simulink library "inp"  (R2021b)
settings: Solver=VariableStepAuto  StartTime=0.0  StopTime=10.0  RelTol=1e-3
undefined symbols (not defined in the file): C_TASK_5MS_S, FALSE, KINP_AcoreReadyToSlp_flg_ovrdflg, KINP_AcoreReadyToSlp_flg_ovrdval, KINP_AllowMovThd_OTA_enum_ovrdflg, KINP_AllowMovThd_OTA_enum_ovrdval, KINP_APSAngleTarget_Deg_ovrdflg, KINP_APSAngleTarget_Deg_ovrdval, KINP_APSDecReq_mps2_ovrdflg, KINP_APSDecReq_mps2_ovrdval, KINP_APSDecReqA_flg_ovrdflg, KINP_APSDecReqA_flg_ovrdval, KINP_APSDFLL_cm_ovrdflg, KINP_APSDFLL_cm_ovrdval, KINP_APSDFLR_cm_ovrdflg, KINP_APSDFLR_cm_ovrdval, KINP_APSDRLL_cm_ovrdflg, KINP_APSDRLL_cm_ovrdval, KINP_APSDRLR_cm_ovrdflg, KINP_APSDRLR_cm_ovrdval, KINP_APSExitCondition_enum_ovrdflg, KINP_APSExitCondition_enum_ovrdval, KINP_APSHWVer_enum_ovrdflg, KINP_APSHWVer_enum_ovrdval, KINP_APSProgressPCT_pct_ovrdflg, KINP_APSProgressPCT_pct_ovrdval, KINP_APSReq_enum_ovrdflg, KINP_APSReq_enum_ovrdval, KINP_APSRQDisplay_enum_ovrdflg, KINP_APSRQDisplay_enum_ovrdval, KINP_APSRqEPASCtrl_flg_ovrdflg, KINP_APSRqEPASCtrl_flg_ovrdval, KINP_APSShiftPosnReq_enum_ovrdval, KINP_APSShiftPosnReq_enum_ovrflg, KINP_APSSpeedCMD_kph_ovrdval, KINP_APSSpeedCMD_kph_ovrflg, KINP_APSStaSystem_enum_ovrdflg, KINP_APSStaSystem_enum_ovrdval, KINP_APSSWVer_enum_ovrdflg, KINP_APSSWVer_enum_ovrdval, KINP_APSVMCReqA_flg_ovrdval, KINP_APSVMCReqA_flg_ovrflg, KINP_APSVRqEPASCtrl_flg_ovrdflg, KINP_APSVRqEPASCtrl_flg_ovrdval, KINP_AuxBattVolmV_mV_ovrdflg, KINP_AuxBattVolmV_mV_ovrdval, KINP_CAASSta_enum_ovrdflg, KINP_CAASSta_enum_ovrdval, KINP_CAASVMCReqA_flg_ovrdval, KINP_CAASVMCReqA_flg_ovrflg, KINP_Chime_enum_ovrdflg, KINP_Chime_enum_ovrdval, KINP_ClearDTCcmd_flg_ovrdflg, KINP_ClearDTCcmd_flg_ovrdval, KINP_EvccAplusPwrUpReq_flg_ovrdflg, KINP_EvccAplusPwrUpReq_flg_ovrdval, KINP_LFID_raw_ovrdval, KINP_LFID_raw_ovrflg, KINP_LRID_raw_ovrdval, KINP_MemOffsetAccX_raw16_ovrdflg ... (+118)
libraries: FVT_lib x942, hcu_lib x1
(part 21 of 31)

== system inp/INP/CAN3/SignalCheck/MCU_N_F1 ==
  BHAL_outputs : Inport
  inp_CanValid_bus : Inport  Port=2
  FrActvDmpDisabStaNidec : FVT_lib/inp/can_signal_template  SystemSampleTime=-1  VariantActivationTime=update diagram  Latency=0  AutoFrameSizeCalculation=off
      link override defval: Value=KINP_FrActvDmpDisabStaNidec_flg_defval
      link override ovrdflg: Value=KINP_FrActvDmpDisabStaNidec_flg_ovrdflg
      link override ovrdval: Value=KINP_FrActvDmpDisabStaNidec_flg_ovrdval
  FrEDUDrtStaNidec : FVT_lib/inp/can_signal_template  SystemSampleTime=-1  VariantActivationTime=update diagram  Latency=0  AutoFrameSizeCalculation=off
      link override defval: Value=KINP_FrEDUDrtStaNidec_flg_defval
      link override ovrdflg: Value=KINP_FrEDUDrtStaNidec_flg_ovrdflg
      link override ovrdval: Value=KINP_FrEDUDrtStaNidec_flg_ovrdval
  FrEDUOpratingStaNidec : FVT_lib/inp/can_signal_template  SystemSampleTime=-1  VariantActivationTime=update diagram  Latency=0  AutoFrameSizeCalculation=off
      link override defval: Value=KINP_FrEDUOpratingStaNidec_flg_defval
      link override ovrdflg: Value=KINP_FrEDUOpratingStaNidec_flg_ovrdflg
      link override ovrdval: Value=KINP_FrEDUOpratingStaNidec_flg_ovrdval
  FrEDURealTMTqNidec : FVT_lib/inp/can_signal_template  SystemSampleTime=-1  VariantActivationTime=update diagram  Latency=0  AutoFrameSizeCalculation=off
      link override defval: Value=KINP_FrEDURealTMTqNidec_Nm_defval
      link override ovrdflg: Value=KINP_FrEDURealTMTqNidec_Nm_ovrdflg
      link override ovrdval: Value=KINP_FrEDURealTMTqNidec_Nm_ovrdval
  FrEDURotateDirctionNidec : FVT_lib/inp/can_signal_template  SystemSampleTime=-1  VariantActivationTime=update diagram  Latency=0  AutoFrameSizeCalculation=off
      link override defval: Value=KINP_FrEDURotateDirctionNidec_enum_defval
      link override ovrdflg: Value=KINP_FrEDURotateDirctionNidec_enum_ovrdflg
      link override ovrdval: Value=KINP_FrEDURotateDirctionNidec_enum_ovrdval
  FrEDUTqReqFbkNidec : FVT_lib/inp/can_signal_template  SystemSampleTime=-1  VariantActivationTime=update diagram  Latency=0  AutoFrameSizeCalculation=off
      link override defval: Value=KINP_FrEDUTqReqFbkNidec_Nm_defval
      link override ovrdflg: Value=KINP_FrEDUTqReqFbkNidec_Nm_ovrdflg
      link override ovrdval: Value=KINP_FrEDUTqReqFbkNidec_Nm_ovrdval
  FrMCU1ChksumNidec : FVT_lib/inp/can_signal_template  SystemSampleTime=-1  VariantActivationTime=update diagram  Latency=0  AutoFrameSizeCalculation=off
      link override defval: Value=KINP_FrMCU1ChksumNidec_enum_defval
      link override ovrdflg: Value=KINP_FrMCU1ChksumNidec_enum_ovrdflg
      link override ovrdval: Value=KINP_FrMCU1ChksumNidec_enum_ovrdval
  FrMCU1RolCntNidec : FVT_lib/inp/can_signal_template  SystemSampleTime=-1  VariantActivationTime=update diagram  Latency=0  AutoFrameSizeCalculation=off
      link override defval: Value=KINP_FrMCU1RolCntNidec_enum_defval
      link override ovrdflg: Value=KINP_FrMCU1RolCntNidec_enum_ovrdflg
      link override ovrdval: Value=KINP_FrMCU1RolCntNidec_enum_ovrdval
  FrMCUBATNidec : FVT_lib/inp/can_signal_template  SystemSampleTime=-1  VariantActivationTime=update diagram  Latency=0  AutoFrameSizeCalculation=off
      link override defval: Value=KINP_FrMCUBATNidec_V_defval
      link override ovrdflg: Value=KINP_FrMCUBATNidec_V_ovrdflg
      link override ovrdval: Value=KINP_FrMCUBATNidec_V_ovrdval
  FrMCUDCBusCurrNidec : FVT_lib/inp/can_signal_template  SystemSampleTime=-1  VariantActivationTime=update diagram  Latency=0  AutoFrameSizeCalculation=off
      link override defval: Value=KINP_FrMCUDCBusCurrNidec_A_defval
      link override ovrdflg: Value=KINP_FrMCUDCBusCurrNidec_A_ovrdflg
      link override ovrdval: Value=KINP_FrMCUDCBusCurrNidec_A_ovrdval
  FrMCUDCBusVoltNidec : FVT_lib/inp/can_signal_template  SystemSampleTime=-1  VariantActivationTime=update diagram  Latency=0  AutoFrameSizeCalculation=off
      link override defval: Value=KINP_FrMCUDCBusVoltNidec_V_defval
      link override ovrdflg: Value=KINP_FrMCUDCBusVoltNidec_V_ovrdflg
      link override ovrdval: Value=KINP_FrMCUDCBusVoltNidec_V_ovrdval
  FrMCUDischrgStaNidec : FVT_lib/inp/can_signal_template  SystemSampleTime=-1  VariantActivationTime=update diagram  Latency=0  AutoFrameSizeCalculation=off
      link override defval: Value=KINP_FrMCUDischrgStaNidec_flg_defval
      link override ovrdflg: Value=KINP_FrMCUDischrgStaNidec_flg_ovrdflg
      link override ovrdval: Value=KINP_FrMCUDischrgStaNidec_flg_ovrdval
  FrMCUEnaStaNidec : FVT_lib/inp/can_signal_template  SystemSampleTime=-1  VariantActivationTime=update diagram  Latency=0  AutoFrameSizeCalculation=off
      link override defval: Value=KINP_FrMCUEnaStaNidec_flg_defval
      link override ovrdflg: Value=KINP_FrMCUEnaStaNidec_flg_ovrdflg
      link override ovrdval: Value=KINP_FrMCUEnaStaNidec_flg_ovrdval
  FrMCUErrNidec : FVT_lib/inp/can_signal_template  SystemSampleTime=-1  VariantActivationTime=update diagram  Latency=0  AutoFrameSizeCalculation=off
      link override defval: Value=KINP_FrMCUErrNidec_enum_defval
      link override ovrdflg: Value=KINP_FrMCUErrNidec_enum_ovrdflg
      link override ovrdval: Value=KINP_FrMCUErrNidec_enum_ovrdval
  FrMCUIGNstaNidec : FVT_lib/inp/can_signal_template  SystemSampleTime=-1  VariantActivationTime=update diagram  Latency=0  AutoFrameSizeCalculation=off
      link override defval: Value=KINP_FrMCUIGNstaNidec_flg_defval
      link override ovrdflg: Value=KINP_FrMCUIGNstaNidec_flg_ovrdflg
      link override ovrdval: Value=KINP_FrMCUIGNstaNidec_flg_ovrdval
  FrMCUReady4PreNidec : FVT_lib/inp/can_signal_template  SystemSampleTime=-1  VariantActivationTime=update diagram  Latency=0  AutoFrameSizeCalculation=off
      link override defval: Value=KINP_FrMCUReady4PreNidec_flg_defval
      link override ovrdflg: Value=KINP_FrMCUReady4PreNidec_flg_ovrdflg
      link override ovrdval: Value=KINP_FrMCUReady4PreNidec_flg_ovrdval
  FrMCUReadyNidec : FVT_lib/inp/can_signal_template  SystemSampleTime=-1  VariantActivationTime=update diagram  Latency=0  AutoFrameSizeCalculation=off
      link override defval: Value=KINP_FrMCUReadyNidec_flg_defval
      link override ovrdflg: Value=KINP_FrMCUReadyNidec_flg_ovrdflg
      link override ovrdval: Value=KINP_FrMCUReadyNidec_flg_ovrdval
  FrMCUSysStaNidec : FVT_lib/inp/can_signal_template  SystemSampleTime=-1  VariantActivationTime=update diagram  Latency=0  AutoFrameSizeCalculation=off
      link override defval: Value=KINP_FrMCUSysStaNidec_enum_defval
      link override ovrdflg: Value=KINP_FrMCUSysStaNidec_enum_ovrdflg
      link override ovrdval: Value=KINP_FrMCUSysStaNidec_enum_ovrdval
  FrMCUTempNidec : FVT_lib/inp/can_signal_template  SystemSampleTime=-1  VariantActivationTime=update diagram  Latency=0  AutoFrameSizeCalculation=off
      link override defval: Value=KINP_FrMCUTempNidec_C_defval
      link override ovrdflg: Value=KINP_FrMCUTempNidec_C_ovrdflg
      link override ovrdval: Value=KINP_FrMCUTempNidec_C_ovrdval
  FrMotorAvailTqNidec : FVT_lib/inp/can_signal_template  SystemSampleTime=-1  VariantActivationTime=update diagram  Latency=0  AutoFrameSizeCalculation=off
      link override defval: Value=KINP_FrMotorAvailTqNidec_Nm_defval
      link override ovrdflg: Value=KINP_FrMotorAvailTqNidec_Nm_ovrdflg
      link override ovrdval: Value=KINP_FrMotorAvailTqNidec_Nm_ovrdval
  FrRegenAvailTqNidec : FVT_lib/inp/can_signal_template  SystemSampleTime=-1  VariantActivationTime=update diagram  Latency=0  AutoFrameSizeCalculation=off
      link override defval: Value=KINP_FrRegenAvailTqNidec_Nm_defval
      link override ovrdflg: Value=KINP_FrRegenAvailTqNidec_Nm_ovrdflg
      link override ovrdval: Value=KINP_FrRegenAvailTqNidec_Nm_ovrdval
  FrTMSpdNidec : FVT_lib/inp/can_signal_template  SystemSampleTime=-1  VariantActivationTime=update diagram  Latency=0  AutoFrameSizeCalculation=off
      link override defval: Value=KINP_FrTMSpdNidec_rpm_defval
      link override ovrdflg: Value=KINP_FrTMSpdNidec_rpm_ovrdflg
      link override ovrdval: Value=KINP_FrTMSpdNidec_rpm_ovrdval
  FrTMTempNidec : FVT_lib/inp/can_signal_template  SystemSampleTime=-1  VariantActivationTime=update diagram  Latency=0  AutoFrameSizeCalculation=off
      link override defval: Value=KINP_FrTMTempNidec_C_defval
      link override ovrdflg: Value=KINP_FrTMTempNidec_C_ovrdflg
      link override ovrdval: Value=KINP_FrTMTempNidec_C_ovrdval
  FrTMidNidec : FVT_lib/inp/can_signal_template  SystemSampleTime=-1  VariantActivationTime=update diagram  Latency=0  AutoFrameSizeCalculation=off
      link override defval: Value=KINP_FrTMidNidec_A_defval
      link override ovrdflg: Value=KINP_FrTMidNidec_A_ovrdflg
      link override ovrdval: Value=KINP_FrTMidNidec_A_ovrdval
  FrTMiqNidec : FVT_lib/inp/can_signal_template  SystemSampleTime=-1  VariantActivationTime=update diagram  Latency=0  AutoFrameSizeCalculation=off
      link override defval: Value=KINP_FrTMiqNidec_A_defval
      link override ovrdflg: Value=KINP_FrTMiqNidec_A_ovrdflg
      link override ovrdval: Value=KINP_FrTMiqNidec_A_ovrdval
  MCUWarnFNidec : FVT_lib/inp/can_signal_template  SystemSampleTime=-1  VariantActivationTime=update diagram  Latency=0  AutoFrameSizeCalculation=off
      link override defval: Value=KINP_MCUWarnFNidec_enum_defval
      link override ovrdflg: Value=KINP_MCUWarnFNidec_enum_ovrdflg
      link override ovrdval: Value=KINP_MCUWarnFNidec_enum_ovrdval
  Terminator_{1..26} (26 alike) : Terminator
  True_VHAL_FrActvDmpDisabStaNidec_flg : Constant  Value=TRUE  OutDataTypeStr=boolean
  True_VHAL_FrEDUDrtStaNidec_flg : Constant  Value=TRUE  OutDataTypeStr=boolean
  True_VHAL_FrEDUOpratingStaNidec_flg : Constant  Value=TRUE  OutDataTypeStr=boolean
  True_VHAL_FrEDURealTMTqNidec_Nm : Constant  Value=TRUE  OutDataTypeStr=boolean
  True_VHAL_FrEDURotateDirctionNidec_enum : Constant  Value=TRUE  OutDataTypeStr=boolean
  True_VHAL_FrEDUTqReqFbkNidec_Nm : Constant  Value=TRUE  OutDataTypeStr=boolean
  True_VHAL_FrMCU1ChksumNidec_enum : Constant  Value=TRUE  OutDataTypeStr=boolean
  True_VHAL_FrMCU1RolCntNidec_enum : Constant  Value=TRUE  OutDataTypeStr=boolean
  True_VHAL_FrMCUBATNidec_V : Constant  Value=TRUE  OutDataTypeStr=boolean
  True_VHAL_FrMCUDCBusCurrNidec_A : Constant  Value=TRUE  OutDataTypeStr=boolean
  True_VHAL_FrMCUDCBusVoltNidec_V : Constant  Value=TRUE  OutDataTypeStr=boolean
  True_VHAL_FrMCUDischrgStaNidec_flg : Constant  Value=TRUE  OutDataTypeStr=boolean
  True_VHAL_FrMCUEnaStaNidec_flg : Constant  Value=TRUE  OutDataTypeStr=boolean
  True_VHAL_FrMCUErrNidec_enum : Constant  Value=TRUE  OutDataTypeStr=boolean
  True_VHAL_FrMCUIGNstaNidec_flg : Constant  Value=TRUE  OutDataTypeStr=boolean
  True_VHAL_FrMCUReady4PreNidec_flg : Constant  Value=TRUE  OutDataTypeStr=boolean
  True_VHAL_FrMCUReadyNidec_flg : Constant  Value=TRUE  OutDataTypeStr=boolean
  True_VHAL_FrMCUSysStaNidec_enum : Constant  Value=TRUE  OutDataTypeStr=boolean
  True_VHAL_FrMCUTempNidec_C : Constant  Value=TRUE  OutDataTypeStr=boolean
  True_VHAL_FrMotorAvailTqNidec_Nm : Constant  Value=TRUE  OutDataTypeStr=boolean
  True_VHAL_FrRegenAvailTqNidec_Nm : Constant  Value=TRUE  OutDataTypeStr=boolean
  True_VHAL_FrTMSpdNidec_rpm : Constant  Value=TRUE  OutDataTypeStr=boolean
  True_VHAL_FrTMTempNidec_C : Constant  Value=TRUE  OutDataTypeStr=boolean
  True_VHAL_FrTMidNidec_A : Constant  Value=TRUE  OutDataTypeStr=boolean
  True_VHAL_FrTMiqNidec_A : Constant  Value=TRUE  OutDataTypeStr=boolean
  True_VHAL_MCUWarnFNidec_enum : Constant  Value=TRUE  OutDataTypeStr=boolean
  slr1_{1..26} (26 alike) : BusSelector  OutputSignals=VINP_CANMsgValidMCUNF1_flg
  slr_VHAL_FrActvDmpDisabStaNidec_flg : BusSelector  OutputSignals=VHAL_FrActvDmpDisabStaNidec_flg
  slr_VHAL_FrEDUDrtStaNidec_flg : BusSelector  OutputSignals=VHAL_FrEDUDrtStaNidec_flg
  slr_VHAL_FrEDUOpratingStaNidec_flg : BusSelector  OutputSignals=VHAL_FrEDUOpratingStaNidec_flg
  slr_VHAL_FrEDURealTMTqNidec_Nm : BusSelector  OutputSignals=VHAL_FrEDURealTMTqNidec_Nm
  slr_VHAL_FrEDURotateDirctionNidec_enum : BusSelector  OutputSignals=VHAL_FrEDURotateDirctionNidec_enum
  slr_VHAL_FrEDUTqReqFbkNidec_Nm : BusSelector  OutputSignals=VHAL_FrEDUTqReqFbkNidec_Nm
  slr_VHAL_FrMCU1ChksumNidec_enum : BusSelector  OutputSignals=VHAL_FrMCU1ChksumNidec_enum
  slr_VHAL_FrMCU1RolCntNidec_enum : BusSelector  OutputSignals=VHAL_FrMCU1RolCntNidec_enum
  slr_VHAL_FrMCUBATNidec_V : BusSelector  OutputSignals=VHAL_FrMCUBATNidec_V
  slr_VHAL_FrMCUDCBusCurrNidec_A : BusSelector  OutputSignals=VHAL_FrMCUDCBusCurrNidec_A
  slr_VHAL_FrMCUDCBusVoltNidec_V : BusSelector  OutputSignals=VHAL_FrMCUDCBusVoltNidec_V
  slr_VHAL_FrMCUDischrgStaNidec_flg : BusSelector  OutputSignals=VHAL_FrMCUDischrgStaNidec_flg
  slr_VHAL_FrMCUEnaStaNidec_flg : BusSelector  OutputSignals=VHAL_FrMCUEnaStaNidec_flg
  slr_VHAL_FrMCUErrNidec_enum : BusSelector  OutputSignals=VHAL_FrMCUErrNidec_enum
  slr_VHAL_FrMCUIGNstaNidec_flg : BusSelector  OutputSignals=VHAL_FrMCUIGNstaNidec_flg
  slr_VHAL_FrMCUReady4PreNidec_flg : BusSelector  OutputSignals=VHAL_FrMCUReady4PreNidec_flg
  slr_VHAL_FrMCUReadyNidec_flg : BusSelector  OutputSignals=VHAL_FrMCUReadyNidec_flg
  slr_VHAL_FrMCUSysStaNidec_enum : BusSelector  OutputSignals=VHAL_FrMCUSysStaNidec_enum
  slr_VHAL_FrMCUTempNidec_C : BusSelector  OutputSignals=VHAL_FrMCUTempNidec_C
  slr_VHAL_FrMotorAvailTqNidec_Nm : BusSelector  OutputSignals=VHAL_FrMotorAvailTqNidec_Nm
  slr_VHAL_FrRegenAvailTqNidec_Nm : BusSelector  OutputSignals=VHAL_FrRegenAvailTqNidec_Nm
  slr_VHAL_FrTMSpdNidec_rpm : BusSelector  OutputSignals=VHAL_FrTMSpdNidec_rpm
  slr_VHAL_FrTMTempNidec_C : BusSelector  OutputSignals=VHAL_FrTMTempNidec_C
  slr_VHAL_FrTMidNidec_A : BusSelector  OutputSignals=VHAL_FrTMidNidec_A
  slr_VHAL_FrTMiqNidec_A : BusSelector  OutputSignals=VHAL_FrTMiqNidec_A
  slr_VHAL_MCUWarnFNidec_enum : BusSelector  OutputSignals=VHAL_MCUWarnFNidec_enum
  VINP_FrActvDmpDisabStaNidec_flg : Outport
  VINP_FrEDUDrtStaNidec_flg : Outport  Port=2
  VINP_FrEDUOpratingStaNidec_flg : Outport  Port=3
  VINP_FrEDURealTMTqNidec_Nm : Outport  Port=4
  VINP_FrEDURotateDirctionNidec_enum : Outport  Port=5
  VINP_FrEDUTqReqFbkNidec_Nm : Outport  Port=6
  VINP_FrMCU1ChksumNidec_enum : Outport  Port=7
  VINP_FrMCU1RolCntNidec_enum : Outport  Port=8
  VINP_FrMCUBATNidec_V : Outport  Port=9
  VINP_FrMCUDCBusCurrNidec_A : Outport  Port=10
  VINP_FrMCUDCBusVoltNidec_V : Outport  Port=11
  VINP_FrMCUDischrgStaNidec_flg : Outport  Port=12
  VINP_FrMCUEnaStaNidec_flg : Outport  Port=13
  VINP_FrMCUErrNidec_enum : Outport  Port=14
  VINP_FrMCUIGNstaNidec_flg : Outport  Port=15
  VINP_FrMCUReady4PreNidec_flg : Outport  Port=16
  VINP_FrMCUReadyNidec_flg : Outport  Port=17
  VINP_FrMCUSysStaNidec_enum : Outport  Port=18
  VINP_FrMCUTempNidec_C : Outport  Port=19
  VINP_FrMotorAvailTqNidec_Nm : Outport  Port=20
  VINP_FrRegenAvailTqNidec_Nm : Outport  Port=21
  VINP_FrTMSpdNidec_rpm : Outport  Port=22
  VINP_FrTMTempNidec_C : Outport  Port=23
  VINP_FrTMidNidec_A : Outport  Port=24
  VINP_FrTMiqNidec_A : Outport  Port=25
  VINP_MCUWarnFNidec_enum : Outport  Port=26
  wires:
  BHAL_outputs/1 -> [BHAL_outputs]
  inp_CanValid_bus/1 -> [inp_CanValid_bus]
  [BHAL_outputs] -> slr_VHAL_FrActvDmpDisabStaNidec_flg/1
  slr_VHAL_FrActvDmpDisabStaNidec_flg/1 -> FrActvDmpDisabStaNidec/1  "<VHAL_FrActvDmpDisabStaNidec_flg>"
  True_VHAL_FrActvDmpDisabStaNidec_flg/1 -> FrActvDmpDisabStaNidec/2
  [inp_CanValid_bus] -> slr1_1/1
  slr1_1/1 -> FrActvDmpDisabStaNidec/3  "<VINP_CANMsgValidMCUNF1_flg>"
  FrActvDmpDisabStaNidec/1 -> VINP_FrActvDmpDisabStaNidec_flg/1  "VINP_FrActvDmpDisabStaNidec_flg"
  FrActvDmpDisabStaNidec/2 -> Terminator_1/1
  [BHAL_outputs] -> slr_VHAL_FrEDUDrtStaNidec_flg/1
  slr_VHAL_FrEDUDrtStaNidec_flg/1 -> FrEDUDrtStaNidec/1  "<VHAL_FrEDUDrtStaNidec_flg>"
  True_VHAL_FrEDUDrtStaNidec_flg/1 -> FrEDUDrtStaNidec/2
  [inp_CanValid_bus] -> slr1_2/1
  slr1_2/1 -> FrEDUDrtStaNidec/3  "<VINP_CANMsgValidMCUNF1_flg>"
  FrEDUDrtStaNidec/1 -> VINP_FrEDUDrtStaNidec_flg/1  "VINP_FrEDUDrtStaNidec_flg"
  FrEDUDrtStaNidec/2 -> Terminator_2/1
  [BHAL_outputs] -> slr_VHAL_FrEDUOpratingStaNidec_flg/1
  slr_VHAL_FrEDUOpratingStaNidec_flg/1 -> FrEDUOpratingStaNidec/1  "<VHAL_FrEDUOpratingStaNidec_flg>"
  True_VHAL_FrEDUOpratingStaNidec_flg/1 -> FrEDUOpratingStaNidec/2
  [inp_CanValid_bus] -> slr1_3/1
  slr1_3/1 -> FrEDUOpratingStaNidec/3  "<VINP_CANMsgValidMCUNF1_flg>"
  FrEDUOpratingStaNidec/1 -> VINP_FrEDUOpratingStaNidec_flg/1  "VINP_FrEDUOpratingStaNidec_flg"
  FrEDUOpratingStaNidec/2 -> Terminator_3/1
  [BHAL_outputs] -> slr_VHAL_FrEDURealTMTqNidec_Nm/1
  slr_VHAL_FrEDURealTMTqNidec_Nm/1 -> FrEDURealTMTqNidec/1  "<VHAL_FrEDURealTMTqNidec_Nm>"
  True_VHAL_FrEDURealTMTqNidec_Nm/1 -> FrEDURealTMTqNidec/2
  [inp_CanValid_bus] -> slr1_4/1
  slr1_4/1 -> FrEDURealTMTqNidec/3  "<VINP_CANMsgValidMCUNF1_flg>"
  FrEDURealTMTqNidec/1 -> VINP_FrEDURealTMTqNidec_Nm/1  "VINP_FrEDURealTMTqNidec_Nm"
  FrEDURealTMTqNidec/2 -> Terminator_4/1
  [BHAL_outputs] -> slr_VHAL_FrEDURotateDirctionNidec_enum/1
  slr_VHAL_FrEDURotateDirctionNidec_enum/1 -> FrEDURotateDirctionNidec/1  "<VHAL_FrEDURotateDirctionNidec_enum>"
  True_VHAL_FrEDURotateDirctionNidec_enum/1 -> FrEDURotateDirctionNidec/2
  [inp_CanValid_bus] -> slr1_5/1
  slr1_5/1 -> FrEDURotateDirctionNidec/3  "<VINP_CANMsgValidMCUNF1_flg>"
  FrEDURotateDirctionNidec/1 -> VINP_FrEDURotateDirctionNidec_enum/1  "VINP_FrEDURotateDirctionNidec_enum"
  FrEDURotateDirctionNidec/2 -> Terminator_5/1
  [BHAL_outputs] -> slr_VHAL_FrEDUTqReqFbkNidec_Nm/1
  slr_VHAL_FrEDUTqReqFbkNidec_Nm/1 -> FrEDUTqReqFbkNidec/1  "<VHAL_FrEDUTqReqFbkNidec_Nm>"
  True_VHAL_FrEDUTqReqFbkNidec_Nm/1 -> FrEDUTqReqFbkNidec/2
  [inp_CanValid_bus] -> slr1_6/1
  slr1_6/1 -> FrEDUTqReqFbkNidec/3  "<VINP_CANMsgValidMCUNF1_flg>"
  FrEDUTqReqFbkNidec/1 -> VINP_FrEDUTqReqFbkNidec_Nm/1  "VINP_FrEDUTqReqFbkNidec_Nm"
  FrEDUTqReqFbkNidec/2 -> Terminator_6/1
  [BHAL_outputs] -> slr_VHAL_FrMCU1ChksumNidec_enum/1
  slr_VHAL_FrMCU1ChksumNidec_enum/1 -> FrMCU1ChksumNidec/1  "<VHAL_FrMCU1ChksumNidec_enum>"
  True_VHAL_FrMCU1ChksumNidec_enum/1 -> FrMCU1ChksumNidec/2
  [inp_CanValid_bus] -> slr1_7/1
  slr1_7/1 -> FrMCU1ChksumNidec/3  "<VINP_CANMsgValidMCUNF1_flg>"
  FrMCU1ChksumNidec/1 -> VINP_FrMCU1ChksumNidec_enum/1  "VINP_FrMCU1ChksumNidec_enum"
  FrMCU1ChksumNidec/2 -> Terminator_7/1
  [BHAL_outputs] -> slr_VHAL_FrMCU1RolCntNidec_enum/1
  slr_VHAL_FrMCU1RolCntNidec_enum/1 -> FrMCU1RolCntNidec/1  "<VHAL_FrMCU1RolCntNidec_enum>"
  True_VHAL_FrMCU1RolCntNidec_enum/1 -> FrMCU1RolCntNidec/2
  [inp_CanValid_bus] -> slr1_8/1
  slr1_8/1 -> FrMCU1RolCntNidec/3  "<VINP_CANMsgValidMCUNF1_flg>"
  FrMCU1RolCntNidec/1 -> VINP_FrMCU1RolCntNidec_enum/1  "VINP_FrMCU1RolCntNidec_enum"
  FrMCU1RolCntNidec/2 -> Terminator_8/1
  [BHAL_outputs] -> slr_VHAL_FrMCUBATNidec_V/1
  slr_VHAL_FrMCUBATNidec_V/1 -> FrMCUBATNidec/1  "<VHAL_FrMCUBATNidec_V>"
  True_VHAL_FrMCUBATNidec_V/1 -> FrMCUBATNidec/2
  [inp_CanValid_bus] -> slr1_9/1
  slr1_9/1 -> FrMCUBATNidec/3  "<VINP_CANMsgValidMCUNF1_flg>"
  FrMCUBATNidec/1 -> VINP_FrMCUBATNidec_V/1  "VINP_FrMCUBATNidec_V"
  FrMCUBATNidec/2 -> Terminator_9/1
  [BHAL_outputs] -> slr_VHAL_FrMCUDCBusCurrNidec_A/1
  slr_VHAL_FrMCUDCBusCurrNidec_A/1 -> FrMCUDCBusCurrNidec/1  "<VHAL_FrMCUDCBusCurrNidec_A>"
  True_VHAL_FrMCUDCBusCurrNidec_A/1 -> FrMCUDCBusCurrNidec/2
  [inp_CanValid_bus] -> slr1_10/1
  slr1_10/1 -> FrMCUDCBusCurrNidec/3  "<VINP_CANMsgValidMCUNF1_flg>"
  FrMCUDCBusCurrNidec/1 -> VINP_FrMCUDCBusCurrNidec_A/1  "VINP_FrMCUDCBusCurrNidec_A"
  FrMCUDCBusCurrNidec/2 -> Terminator_10/1
  [BHAL_outputs] -> slr_VHAL_FrMCUDCBusVoltNidec_V/1
  slr_VHAL_FrMCUDCBusVoltNidec_V/1 -> FrMCUDCBusVoltNidec/1  "<VHAL_FrMCUDCBusVoltNidec_V>"
  True_VHAL_FrMCUDCBusVoltNidec_V/1 -> FrMCUDCBusVoltNidec/2
  [inp_CanValid_bus] -> slr1_11/1
  slr1_11/1 -> FrMCUDCBusVoltNidec/3  "<VINP_CANMsgValidMCUNF1_flg>"
  FrMCUDCBusVoltNidec/1 -> VINP_FrMCUDCBusVoltNidec_V/1  "VINP_FrMCUDCBusVoltNidec_V"
  FrMCUDCBusVoltNidec/2 -> Terminator_11/1
  [BHAL_outputs] -> slr_VHAL_FrMCUDischrgStaNidec_flg/1
  slr_VHAL_FrMCUDischrgStaNidec_flg/1 -> FrMCUDischrgStaNidec/1  "<VHAL_FrMCUDischrgStaNidec_flg>"
  True_VHAL_FrMCUDischrgStaNidec_flg/1 -> FrMCUDischrgStaNidec/2
  [inp_CanValid_bus] -> slr1_12/1
  slr1_12/1 -> FrMCUDischrgStaNidec/3  "<VINP_CANMsgValidMCUNF1_flg>"
  FrMCUDischrgStaNidec/1 -> VINP_FrMCUDischrgStaNidec_flg/1  "VINP_FrMCUDischrgStaNidec_flg"
  FrMCUDischrgStaNidec/2 -> Terminator_12/1
  [BHAL_outputs] -> slr_VHAL_FrMCUEnaStaNidec_flg/1
  slr_VHAL_FrMCUEnaStaNidec_flg/1 -> FrMCUEnaStaNidec/1  "<VHAL_FrMCUEnaStaNidec_flg>"
  True_VHAL_FrMCUEnaStaNidec_flg/1 -> FrMCUEnaStaNidec/2
  [inp_CanValid_bus] -> slr1_13/1
  slr1_13/1 -> FrMCUEnaStaNidec/3  "<VINP_CANMsgValidMCUNF1_flg>"
  FrMCUEnaStaNidec/1 -> VINP_FrMCUEnaStaNidec_flg/1  "VINP_FrMCUEnaStaNidec_flg"
  FrMCUEnaStaNidec/2 -> Terminator_13/1
  [BHAL_outputs] -> slr_VHAL_FrMCUErrNidec_enum/1
  slr_VHAL_FrMCUErrNidec_enum/1 -> FrMCUErrNidec/1  "<VHAL_FrMCUErrNidec_enum>"
  True_VHAL_FrMCUErrNidec_enum/1 -> FrMCUErrNidec/2
  [inp_CanValid_bus] -> slr1_14/1
  slr1_14/1 -> FrMCUErrNidec/3  "<VINP_CANMsgValidMCUNF1_flg>"
  FrMCUErrNidec/1 -> VINP_FrMCUErrNidec_enum/1  "VINP_FrMCUErrNidec_enum"
  FrMCUErrNidec/2 -> Terminator_14/1
  [BHAL_outputs] -> slr_VHAL_FrMCUIGNstaNidec_flg/1
  slr_VHAL_FrMCUIGNstaNidec_flg/1 -> FrMCUIGNstaNidec/1  "<VHAL_FrMCUIGNstaNidec_flg>"
  True_VHAL_FrMCUIGNstaNidec_flg/1 -> FrMCUIGNstaNidec/2
  [inp_CanValid_bus] -> slr1_15/1
  slr1_15/1 -> FrMCUIGNstaNidec/3  "<VINP_CANMsgValidMCUNF1_flg>"
  FrMCUIGNstaNidec/1 -> VINP_FrMCUIGNstaNidec_flg/1  "VINP_FrMCUIGNstaNidec_flg"
  FrMCUIGNstaNidec/2 -> Terminator_15/1
  [BHAL_outputs] -> slr_VHAL_FrMCUReady4PreNidec_flg/1
  slr_VHAL_FrMCUReady4PreNidec_flg/1 -> FrMCUReady4PreNidec/1  "<VHAL_FrMCUReady4PreNidec_flg>"
  True_VHAL_FrMCUReady4PreNidec_flg/1 -> FrMCUReady4PreNidec/2
  [inp_CanValid_bus] -> slr1_16/1
  slr1_16/1 -> FrMCUReady4PreNidec/3  "<VINP_CANMsgValidMCUNF1_flg>"
  FrMCUReady4PreNidec/1 -> VINP_FrMCUReady4PreNidec_flg/1  "VINP_FrMCUReady4PreNidec_flg"
  FrMCUReady4PreNidec/2 -> Terminator_16/1
  [BHAL_outputs] -> slr_VHAL_FrMCUReadyNidec_flg/1
  slr_VHAL_FrMCUReadyNidec_flg/1 -> FrMCUReadyNidec/1  "<VHAL_FrMCUReadyNidec_flg>"
  True_VHAL_FrMCUReadyNidec_flg/1 -> FrMCUReadyNidec/2
  [inp_CanValid_bus] -> slr1_17/1
  slr1_17/1 -> FrMCUReadyNidec/3  "<VINP_CANMsgValidMCUNF1_flg>"
  FrMCUReadyNidec/1 -> VINP_FrMCUReadyNidec_flg/1  "VINP_FrMCUReadyNidec_flg"
  FrMCUReadyNidec/2 -> Terminator_17/1
  [BHAL_outputs] -> slr_VHAL_FrMCUSysStaNidec_enum/1
  slr_VHAL_FrMCUSysStaNidec_enum/1 -> FrMCUSysStaNidec/1  "<VHAL_FrMCUSysStaNidec_enum>"
  True_VHAL_FrMCUSysStaNidec_enum/1 -> FrMCUSysStaNidec/2
  [inp_CanValid_bus] -> slr1_18/1
  slr1_18/1 -> FrMCUSysStaNidec/3  "<VINP_CANMsgValidMCUNF1_flg>"
  FrMCUSysStaNidec/1 -> VINP_FrMCUSysStaNidec_enum/1  "VINP_FrMCUSysStaNidec_enum"
  FrMCUSysStaNidec/2 -> Terminator_18/1
  [BHAL_outputs] -> slr_VHAL_FrMCUTempNidec_C/1
  slr_VHAL_FrMCUTempNidec_C/1 -> FrMCUTempNidec/1  "<VHAL_FrMCUTempNidec_C>"
  True_VHAL_FrMCUTempNidec_C/1 -> FrMCUTempNidec/2
  [inp_CanValid_bus] -> slr1_19/1
  slr1_19/1 -> FrMCUTempNidec/3  "<VINP_CANMsgValidMCUNF1_flg>"
  FrMCUTempNidec/1 -> VINP_FrMCUTempNidec_C/1  "VINP_FrMCUTempNidec_C"
  FrMCUTempNidec/2 -> Terminator_19/1
  [BHAL_outputs] -> slr_VHAL_FrMotorAvailTqNidec_Nm/1
  slr_VHAL_FrMotorAvailTqNidec_Nm/1 -> FrMotorAvailTqNidec/1  "<VHAL_FrMotorAvailTqNidec_Nm>"
  True_VHAL_FrMotorAvailTqNidec_Nm/1 -> FrMotorAvailTqNidec/2
  [inp_CanValid_bus] -> slr1_20/1
  slr1_20/1 -> FrMotorAvailTqNidec/3  "<VINP_CANMsgValidMCUNF1_flg>"
  FrMotorAvailTqNidec/1 -> VINP_FrMotorAvailTqNidec_Nm/1  "VINP_FrMotorAvailTqNidec_Nm"
  FrMotorAvailTqNidec/2 -> Terminator_20/1
  [BHAL_outputs] -> slr_VHAL_FrRegenAvailTqNidec_Nm/1
  slr_VHAL_FrRegenAvailTqNidec_Nm/1 -> FrRegenAvailTqNidec/1  "<VHAL_FrRegenAvailTqNidec_Nm>"
  True_VHAL_FrRegenAvailTqNidec_Nm/1 -> FrRegenAvailTqNidec/2
  [inp_CanValid_bus] -> slr1_21/1
  slr1_21/1 -> FrRegenAvailTqNidec/3  "<VINP_CANMsgValidMCUNF1_flg>"
  FrRegenAvailTqNidec/1 -> VINP_FrRegenAvailTqNidec_Nm/1  "VINP_FrRegenAvailTqNidec_Nm"
  FrRegenAvailTqNidec/2 -> Terminator_21/1
  [BHAL_outputs] -> slr_VHAL_FrTMSpdNidec_rpm/1
  slr_VHAL_FrTMSpdNidec_rpm/1 -> FrTMSpdNidec/1  "<VHAL_FrTMSpdNidec_rpm>"
  True_VHAL_FrTMSpdNidec_rpm/1 -> FrTMSpdNidec/2
  [inp_CanValid_bus] -> slr1_22/1
  slr1_22/1 -> FrTMSpdNidec/3  "<VINP_CANMsgValidMCUNF1_flg>"
  FrTMSpdNidec/1 -> VINP_FrTMSpdNidec_rpm/1  "VINP_FrTMSpdNidec_rpm"
  FrTMSpdNidec/2 -> Terminator_22/1
  [BHAL_outputs] -> slr_VHAL_FrTMTempNidec_C/1
  slr_VHAL_FrTMTempNidec_C/1 -> FrTMTempNidec/1  "<VHAL_FrTMTempNidec_C>"
  True_VHAL_FrTMTempNidec_C/1 -> FrTMTempNidec/2
  [inp_CanValid_bus] -> slr1_23/1
  slr1_23/1 -> FrTMTempNidec/3  "<VINP_CANMsgValidMCUNF1_flg>"
  FrTMTempNidec/1 -> VINP_FrTMTempNidec_C/1  "VINP_FrTMTempNidec_C"
  FrTMTempNidec/2 -> Terminator_23/1
  [BHAL_outputs] -> slr_VHAL_FrTMidNidec_A/1
  slr_VHAL_FrTMidNidec_A/1 -> FrTMidNidec/1  "<VHAL_FrTMidNidec_A>"
  True_VHAL_FrTMidNidec_A/1 -> FrTMidNidec/2
  [inp_CanValid_bus] -> slr1_24/1
  slr1_24/1 -> FrTMidNidec/3  "<VINP_CANMsgValidMCUNF1_flg>"
  FrTMidNidec/1 -> VINP_FrTMidNidec_A/1  "VINP_FrTMidNidec_A"
  FrTMidNidec/2 -> Terminator_24/1
  [BHAL_outputs] -> slr_VHAL_FrTMiqNidec_A/1
  slr_VHAL_FrTMiqNidec_A/1 -> FrTMiqNidec/1  "<VHAL_FrTMiqNidec_A>"
  True_VHAL_FrTMiqNidec_A/1 -> FrTMiqNidec/2
  [inp_CanValid_bus] -> slr1_25/1
  slr1_25/1 -> FrTMiqNidec/3  "<VINP_CANMsgValidMCUNF1_flg>"
  FrTMiqNidec/1 -> VINP_FrTMiqNidec_A/1  "VINP_FrTMiqNidec_A"
  FrTMiqNidec/2 -> Terminator_25/1
  [BHAL_outputs] -> slr_VHAL_MCUWarnFNidec_enum/1
  slr_VHAL_MCUWarnFNidec_enum/1 -> MCUWarnFNidec/1  "<VHAL_MCUWarnFNidec_enum>"
  True_VHAL_MCUWarnFNidec_enum/1 -> MCUWarnFNidec/2
  [inp_CanValid_bus] -> slr1_26/1
  slr1_26/1 -> MCUWarnFNidec/3  "<VINP_CANMsgValidMCUNF1_flg>"
  MCUWarnFNidec/1 -> VINP_MCUWarnFNidec_enum/1  "VINP_MCUWarnFNidec_enum"
  MCUWarnFNidec/2 -> Terminator_26/1

== system inp/INP/CAN3/SignalCheck/MCU_N_F2 ==
  BHAL_outputs : Inport
  inp_CanValid_bus : Inport  Port=2
  FrCoolanttempReqNidec : FVT_lib/inp/can_signal_template  SystemSampleTime=-1  VariantActivationTime=update diagram  Latency=0  AutoFrameSizeCalculation=off
      link override defval: Value=KINP_FrCoolanttempReqNidec_C_defval
      link override ovrdflg: Value=KINP_FrCoolanttempReqNidec_C_ovrdflg
      link override ovrdval: Value=KINP_FrCoolanttempReqNidec_C_ovrdval
  FrEOPSpdSetNidec : FVT_lib/inp/can_signal_template  SystemSampleTime=-1  VariantActivationTime=update diagram  Latency=0  AutoFrameSizeCalculation=off
      link override defval: Value=KINP_FrEOPSpdSetNidec_rpm_defval
      link override ovrdflg: Value=KINP_FrEOPSpdSetNidec_rpm_ovrdflg
      link override ovrdval: Value=KINP_FrEOPSpdSetNidec_rpm_ovrdval
  FrFailcode1Nidec : FVT_lib/inp/can_signal_template  SystemSampleTime=-1  VariantActivationTime=update diagram  Latency=0  AutoFrameSizeCalculation=off
      link override defval: Value=KINP_FrFailcode1Nidec_enum_defval
      link override ovrdflg: Value=KINP_FrFailcode1Nidec_enum_ovrdflg
      link override ovrdval: Value=KINP_FrFailcode1Nidec_enum_ovrdval
  FrFailcode2Nidec : FVT_lib/inp/can_signal_template  SystemSampleTime=-1  VariantActivationTime=update diagram  Latency=0  AutoFrameSizeCalculation=off
      link override defval: Value=KINP_FrFailcode2Nidec_enum_defval
      link override ovrdflg: Value=KINP_FrFailcode2Nidec_enum_ovrdflg
      link override ovrdval: Value=KINP_FrFailcode2Nidec_enum_ovrdval
  FrFailcodehistory1Nidec : FVT_lib/inp/can_signal_template  SystemSampleTime=-1  VariantActivationTime=update diagram  Latency=0  AutoFrameSizeCalculation=off
      link override defval: Value=KINP_FrFailcodehistory1Nidec_enum_defval
      link override ovrdflg: Value=KINP_FrFailcodehistory1Nidec_enum_ovrdflg
      link override ovrdval: Value=KINP_FrFailcodehistory1Nidec_enum_ovrdval
  FrFailcodehistory2Nidec : FVT_lib/inp/can_signal_template  SystemSampleTime=-1  VariantActivationTime=update diagram  Latency=0  AutoFrameSizeCalculation=off
      link override defval: Value=KINP_FrFailcodehistory2Nidec_enum_defval
      link override ovrdflg: Value=KINP_FrFailcodehistory2Nidec_enum_ovrdflg
      link override ovrdval: Value=KINP_FrFailcodehistory2Nidec_enum_ovrdval
  FrLLCTempNidec : FVT_lib/inp/can_signal_template  SystemSampleTime=-1  VariantActivationTime=update diagram  Latency=0  AutoFrameSizeCalculation=off
      link override defval: Value=KINP_FrLLCTempNidec_C_defval
      link override ovrdflg: Value=KINP_FrLLCTempNidec_C_ovrdflg
      link override ovrdval: Value=KINP_FrLLCTempNidec_C_ovrdval
  FrLLCflowReqNidec : FVT_lib/inp/can_signal_template  SystemSampleTime=-1  VariantActivationTime=update diagram  Latency=0  AutoFrameSizeCalculation=off
      link override defval: Value=KINP_FrLLCflowReqNidec_Lpmin_defval
      link override ovrdflg: Value=KINP_FrLLCflowReqNidec_Lpmin_ovrdflg
      link override ovrdval: Value=KINP_FrLLCflowReqNidec_Lpmin_ovrdval
  FrMCUTempWarnNidec : FVT_lib/inp/can_signal_template  SystemSampleTime=-1  VariantActivationTime=update diagram  Latency=0  AutoFrameSizeCalculation=off
      link override defval: Value=KINP_FrMCUTempWarnNidec_enum_defval
      link override ovrdflg: Value=KINP_FrMCUTempWarnNidec_enum_ovrdflg
      link override ovrdval: Value=KINP_FrMCUTempWarnNidec_enum_ovrdval
  FrTMTempWarnNidec : FVT_lib/inp/can_signal_template  SystemSampleTime=-1  VariantActivationTime=update diagram  Latency=0  AutoFrameSizeCalculation=off
      link override defval: Value=KINP_FrTMTempWarnNidec_enum_defval
      link override ovrdflg: Value=KINP_FrTMTempWarnNidec_enum_ovrdflg
      link override ovrdval: Value=KINP_FrTMTempWarnNidec_enum_ovrdval
  Terminator_{1..10} (10 alike) : Terminator
  True_VHAL_FrCoolanttempReqNidec_C : Constant  Value=TRUE  OutDataTypeStr=boolean
  True_VHAL_FrEOPSpdSetNidec_rpm : Constant  Value=TRUE  OutDataTypeStr=boolean
  True_VHAL_FrFailcode1Nidec_enum : Constant  Value=TRUE  OutDataTypeStr=boolean
  True_VHAL_FrFailcode2Nidec_enum : Constant  Value=TRUE  OutDataTypeStr=boolean
  True_VHAL_FrFailcodehistory1Nidec_enum : Constant  Value=TRUE  OutDataTypeStr=boolean
  True_VHAL_FrFailcodehistory2Nidec_enum : Constant  Value=TRUE  OutDataTypeStr=boolean
  True_VHAL_FrLLCTempNidec_C : Constant  Value=TRUE  OutDataTypeStr=boolean
  True_VHAL_FrLLCflowReqNidec_Lpmin : Constant  Value=TRUE  OutDataTypeStr=boolean
  True_VHAL_FrMCUTempWarnNidec_enum : Constant  Value=TRUE  OutDataTypeStr=boolean
  True_VHAL_FrTMTempWarnNidec_enum : Constant  Value=TRUE  OutDataTypeStr=boolean
  slr1_{1..10} (10 alike) : BusSelector  OutputSignals=VINP_CANMsgValidMCUNF2_flg
  slr_VHAL_FrCoolanttempReqNidec_C : BusSelector  OutputSignals=VHAL_FrCoolanttempReqNidec_C
  slr_VHAL_FrEOPSpdSetNidec_rpm : BusSelector  OutputSignals=VHAL_FrEOPSpdSetNidec_rpm
  slr_VHAL_FrFailcode1Nidec_enum : BusSelector  OutputSignals=VHAL_FrFailcode1Nidec_enum
  slr_VHAL_FrFailcode2Nidec_enum : BusSelector  OutputSignals=VHAL_FrFailcode2Nidec_enum
  slr_VHAL_FrFailcodehistory1Nidec_enum : BusSelector  OutputSignals=VHAL_FrFailcodehistory1Nidec_enum
  slr_VHAL_FrFailcodehistory2Nidec_enum : BusSelector  OutputSignals=VHAL_FrFailcodehistory2Nidec_enum
  slr_VHAL_FrLLCTempNidec_C : BusSelector  OutputSignals=VHAL_FrLLCTempNidec_C
  slr_VHAL_FrLLCflowReqNidec_Lpmin : BusSelector  OutputSignals=VHAL_FrLLCflowReqNidec_Lpmin
  slr_VHAL_FrMCUTempWarnNidec_enum : BusSelector  OutputSignals=VHAL_FrMCUTempWarnNidec_enum
  slr_VHAL_FrTMTempWarnNidec_enum : BusSelector  OutputSignals=VHAL_FrTMTempWarnNidec_enum
  VINP_FrCoolanttempReqNidec_C : Outport
  VINP_FrEOPSpdSetNidec_rpm : Outport  Port=2
  VINP_FrFailcode1Nidec_enum : Outport  Port=3
  VINP_FrFailcode2Nidec_enum : Outport  Port=4
  VINP_FrFailcodehistory1Nidec_enum : Outport  Port=5
  VINP_FrFailcodehistory2Nidec_enum : Outport  Port=6
  VINP_FrLLCTempNidec_C : Outport  Port=7
  VINP_FrLLCflowReqNidec_Lpmin : Outport  Port=8
  VINP_FrMCUTempWarnNidec_enum : Outport  Port=9
  VINP_FrTMTempWarnNidec_enum : Outport  Port=10
  wires:
  BHAL_outputs/1 -> [BHAL_outputs]
  inp_CanValid_bus/1 -> [inp_CanValid_bus]
  [BHAL_outputs] -> slr_VHAL_FrCoolanttempReqNidec_C/1
  slr_VHAL_FrCoolanttempReqNidec_C/1 -> FrCoolanttempReqNidec/1  "<VHAL_FrCoolanttempReqNidec_C>"
  True_VHAL_FrCoolanttempReqNidec_C/1 -> FrCoolanttempReqNidec/2
  [inp_CanValid_bus] -> slr1_1/1
  slr1_1/1 -> FrCoolanttempReqNidec/3  "<VINP_CANMsgValidMCUNF2_flg>"
  FrCoolanttempReqNidec/1 -> VINP_FrCoolanttempReqNidec_C/1  "VINP_FrCoolanttempReqNidec_C"
  FrCoolanttempReqNidec/2 -> Terminator_1/1
  [BHAL_outputs] -> slr_VHAL_FrEOPSpdSetNidec_rpm/1
  slr_VHAL_FrEOPSpdSetNidec_rpm/1 -> FrEOPSpdSetNidec/1  "<VHAL_FrEOPSpdSetNidec_rpm>"
  True_VHAL_FrEOPSpdSetNidec_rpm/1 -> FrEOPSpdSetNidec/2
  [inp_CanValid_bus] -> slr1_2/1
  slr1_2/1 -> FrEOPSpdSetNidec/3  "<VINP_CANMsgValidMCUNF2_flg>"
  FrEOPSpdSetNidec/1 -> VINP_FrEOPSpdSetNidec_rpm/1  "VINP_FrEOPSpdSetNidec_rpm"
  FrEOPSpdSetNidec/2 -> Terminator_2/1
  [BHAL_outputs] -> slr_VHAL_FrFailcode1Nidec_enum/1
  slr_VHAL_FrFailcode1Nidec_enum/1 -> FrFailcode1Nidec/1  "<VHAL_FrFailcode1Nidec_enum>"
  True_VHAL_FrFailcode1Nidec_enum/1 -> FrFailcode1Nidec/2
  [inp_CanValid_bus] -> slr1_3/1
  slr1_3/1 -> FrFailcode1Nidec/3  "<VINP_CANMsgValidMCUNF2_flg>"
  FrFailcode1Nidec/1 -> VINP_FrFailcode1Nidec_enum/1  "VINP_FrFailcode1Nidec_enum"
  FrFailcode1Nidec/2 -> Terminator_3/1
  [BHAL_outputs] -> slr_VHAL_FrFailcode2Nidec_enum/1
  slr_VHAL_FrFailcode2Nidec_enum/1 -> FrFailcode2Nidec/1  "<VHAL_FrFailcode2Nidec_enum>"
  True_VHAL_FrFailcode2Nidec_enum/1 -> FrFailcode2Nidec/2
  [inp_CanValid_bus] -> slr1_4/1
  slr1_4/1 -> FrFailcode2Nidec/3  "<VINP_CANMsgValidMCUNF2_flg>"
  FrFailcode2Nidec/1 -> VINP_FrFailcode2Nidec_enum/1  "VINP_FrFailcode2Nidec_enum"
  FrFailcode2Nidec/2 -> Terminator_4/1
  [BHAL_outputs] -> slr_VHAL_FrFailcodehistory1Nidec_enum/1
  slr_VHAL_FrFailcodehistory1Nidec_enum/1 -> FrFailcodehistory1Nidec/1  "<VHAL_FrFailcodehistory1Nidec_enum>"
  True_VHAL_FrFailcodehistory1Nidec_enum/1 -> FrFailcodehistory1Nidec/2
  [inp_CanValid_bus] -> slr1_5/1
  slr1_5/1 -> FrFailcodehistory1Nidec/3  "<VINP_CANMsgValidMCUNF2_flg>"
  FrFailcodehistory1Nidec/1 -> VINP_FrFailcodehistory1Nidec_enum/1  "VINP_FrFailcodehistory1Nidec_enum"
  FrFailcodehistory1Nidec/2 -> Terminator_5/1
  [BHAL_outputs] -> slr_VHAL_FrFailcodehistory2Nidec_enum/1
  slr_VHAL_FrFailcodehistory2Nidec_enum/1 -> FrFailcodehistory2Nidec/1  "<VHAL_FrFailcodehistory2Nidec_enum>"
  True_VHAL_FrFailcodehistory2Nidec_enum/1 -> FrFailcodehistory2Nidec/2
  [inp_CanValid_bus] -> slr1_6/1
  slr1_6/1 -> FrFailcodehistory2Nidec/3  "<VINP_CANMsgValidMCUNF2_flg>"
  FrFailcodehistory2Nidec/1 -> VINP_FrFailcodehistory2Nidec_enum/1  "VINP_FrFailcodehistory2Nidec_enum"
  FrFailcodehistory2Nidec/2 -> Terminator_6/1
  [BHAL_outputs] -> slr_VHAL_FrLLCTempNidec_C/1
  slr_VHAL_FrLLCTempNidec_C/1 -> FrLLCTempNidec/1  "<VHAL_FrLLCTempNidec_C>"
  True_VHAL_FrLLCTempNidec_C/1 -> FrLLCTempNidec/2
  [inp_CanValid_bus] -> slr1_7/1
  slr1_7/1 -> FrLLCTempNidec/3  "<VINP_CANMsgValidMCUNF2_flg>"
  FrLLCTempNidec/1 -> VINP_FrLLCTempNidec_C/1  "VINP_FrLLCTempNidec_C"
  FrLLCTempNidec/2 -> Terminator_7/1
  [BHAL_outputs] -> slr_VHAL_FrLLCflowReqNidec_Lpmin/1
  slr_VHAL_FrLLCflowReqNidec_Lpmin/1 -> FrLLCflowReqNidec/1  "<VHAL_FrLLCflowReqNidec_Lpmin>"
  True_VHAL_FrLLCflowReqNidec_Lpmin/1 -> FrLLCflowReqNidec/2
  [inp_CanValid_bus] -> slr1_8/1
  slr1_8/1 -> FrLLCflowReqNidec/3  "<VINP_CANMsgValidMCUNF2_flg>"
  FrLLCflowReqNidec/1 -> VINP_FrLLCflowReqNidec_Lpmin/1  "VINP_FrLLCflowReqNidec_Lpmin"
  FrLLCflowReqNidec/2 -> Terminator_8/1
  [BHAL_outputs] -> slr_VHAL_FrMCUTempWarnNidec_enum/1
  slr_VHAL_FrMCUTempWarnNidec_enum/1 -> FrMCUTempWarnNidec/1  "<VHAL_FrMCUTempWarnNidec_enum>"
  True_VHAL_FrMCUTempWarnNidec_enum/1 -> FrMCUTempWarnNidec/2
  [inp_CanValid_bus] -> slr1_9/1
  slr1_9/1 -> FrMCUTempWarnNidec/3  "<VINP_CANMsgValidMCUNF2_flg>"
  FrMCUTempWarnNidec/1 -> VINP_FrMCUTempWarnNidec_enum/1  "VINP_FrMCUTempWarnNidec_enum"
  FrMCUTempWarnNidec/2 -> Terminator_9/1
  [BHAL_outputs] -> slr_VHAL_FrTMTempWarnNidec_enum/1
  slr_VHAL_FrTMTempWarnNidec_enum/1 -> FrTMTempWarnNidec/1  "<VHAL_FrTMTempWarnNidec_enum>"
  True_VHAL_FrTMTempWarnNidec_enum/1 -> FrTMTempWarnNidec/2
  [inp_CanValid_bus] -> slr1_10/1
  slr1_10/1 -> FrTMTempWarnNidec/3  "<VINP_CANMsgValidMCUNF2_flg>"
  FrTMTempWarnNidec/1 -> VINP_FrTMTempWarnNidec_enum/1  "VINP_FrTMTempWarnNidec_enum"
  FrTMTempWarnNidec/2 -> Terminator_10/1

== system inp/INP/CAN3/SignalCheck/MCU_N_F3 ==
  BHAL_outputs : Inport
  inp_CanValid_bus : Inport  Port=2
  FrMCUHWVerNidec : FVT_lib/inp/can_signal_template  SystemSampleTime=-1  VariantActivationTime=update diagram  Latency=0  AutoFrameSizeCalculation=off
      link override defval: Value=KINP_FrMCUHWVerNidec_enum_defval
      link override ovrdflg: Value=KINP_FrMCUHWVerNidec_enum_ovrdflg
      link override ovrdval: Value=KINP_FrMCUHWVerNidec_enum_ovrdval
  FrMCUSWVerNidec : FVT_lib/inp/can_signal_template  SystemSampleTime=-1  VariantActivationTime=update diagram  Latency=0  AutoFrameSizeCalculation=off
      link override defval: Value=KINP_FrMCUSWVerNidec_enum_defval
      link override ovrdflg: Value=KINP_FrMCUSWVerNidec_enum_ovrdflg
      link override ovrdval: Value=KINP_FrMCUSWVerNidec_enum_ovrdval
  Terminator_1 : Terminator
  Terminator_2 : Terminator
  True_VHAL_FrMCUHWVerNidec_enum : Constant  Value=TRUE  OutDataTypeStr=boolean
  True_VHAL_FrMCUSWVerNidec_enum : Constant  Value=TRUE  OutDataTypeStr=boolean
  slr1_1 : BusSelector  OutputSignals=VINP_CANMsgValidMCUNF3_flg
  slr1_2 : BusSelector  OutputSignals=VINP_CANMsgValidMCUNF3_flg
  slr_VHAL_FrMCUHWVerNidec_enum : BusSelector  OutputSignals=VHAL_FrMCUHWVerNidec_enum
  slr_VHAL_FrMCUSWVerNidec_enum : BusSelector  OutputSignals=VHAL_FrMCUSWVerNidec_enum
  VINP_FrMCUHWVerNidec_enum : Outport
  VINP_FrMCUSWVerNidec_enum : Outport  Port=2
  wires:
  BHAL_outputs/1 -> [BHAL_outputs]
  inp_CanValid_bus/1 -> [inp_CanValid_bus]
  [BHAL_outputs] -> slr_VHAL_FrMCUHWVerNidec_enum/1
  slr_VHAL_FrMCUHWVerNidec_enum/1 -> FrMCUHWVerNidec/1  "<VHAL_FrMCUHWVerNidec_enum>"
  True_VHAL_FrMCUHWVerNidec_enum/1 -> FrMCUHWVerNidec/2
  [inp_CanValid_bus] -> slr1_1/1
  slr1_1/1 -> FrMCUHWVerNidec/3  "<VINP_CANMsgValidMCUNF3_flg>"
  FrMCUHWVerNidec/1 -> VINP_FrMCUHWVerNidec_enum/1  "VINP_FrMCUHWVerNidec_enum"
  FrMCUHWVerNidec/2 -> Terminator_1/1
  [BHAL_outputs] -> slr_VHAL_FrMCUSWVerNidec_enum/1
  slr_VHAL_FrMCUSWVerNidec_enum/1 -> FrMCUSWVerNidec/1  "<VHAL_FrMCUSWVerNidec_enum>"
  True_VHAL_FrMCUSWVerNidec_enum/1 -> FrMCUSWVerNidec/2
  [inp_CanValid_bus] -> slr1_2/1
  slr1_2/1 -> FrMCUSWVerNidec/3  "<VINP_CANMsgValidMCUNF3_flg>"
  FrMCUSWVerNidec/1 -> VINP_FrMCUSWVerNidec_enum/1  "VINP_FrMCUSWVerNidec_enum"
  FrMCUSWVerNidec/2 -> Terminator_2/1
